simulink model "model_report_gutman"  (R2018b)
settings: Solver=FixedStepAuto  StartTime=0.0  StopTime=10  FixedStep=Ts/100  RelTol=1e-3
StopFcn:
  | %figure;plot(true_position.Data(:,1),true_position.Data(:,2))
values from neighbouring files (symbols this model uses):
  b = 1.115    [report_gutman.m]
  bike_params = [g h b a lambda m]    [report_gutman.m]
  IMU_height = 0.45    [report_gutman.m]
  initial_roll = deg2rad(2)    [report_gutman.m]
  initial_rollrate = deg2rad(2)    [report_gutman.m]
  lambda = deg2rad(90-24)    [report_gutman.m]
  num_tf_steering = [253.4]    [report_gutman.m]
  Ts = 0.01    [report_gutman.m]
  v = 4    [report_gutman.m]
undefined symbols (not defined in the file or in its folder): A, B, C, D, lqr_gains, velocity_lqr
libraries: simulink_extras x6, simulink x1
settings Model: Creator=maximef  LastModifiedBy=maximef

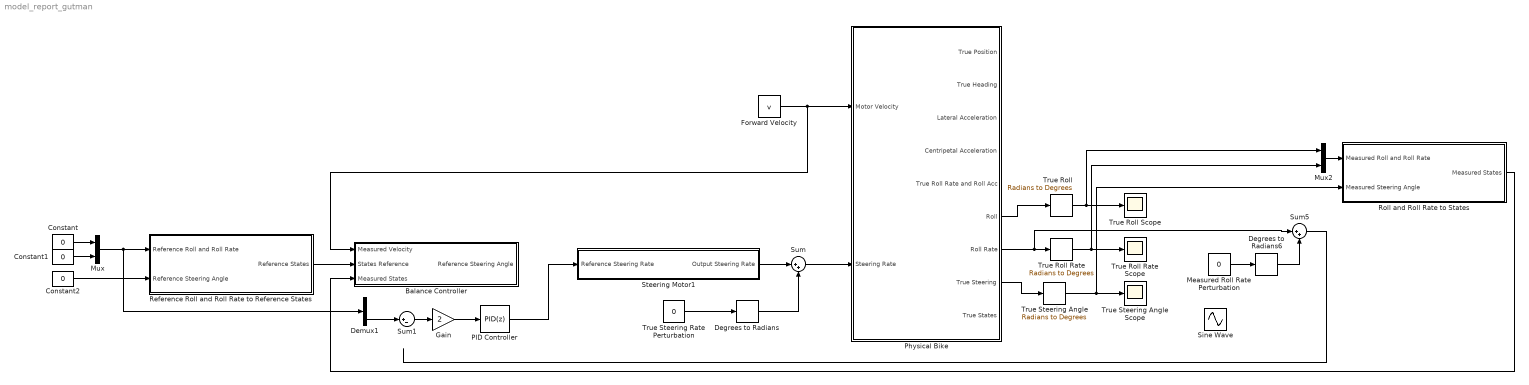
== system model_report_gutman ==
  Balance Controller : Subsystem  SystemSampleTime=Ts
  Constant : Constant  Value=0
  Constant1 : Constant  Value=0
  Constant2 : Constant  Value=0
  Degrees to Radians : simulink_extras/Transformations/Degrees to Radians
  Degrees to Radians6 : simulink_extras/Transformations/Degrees to Radians
  Demux1 : Demux  Outputs=2
  Forward Velocity : Constant  Value=v
  Gain : Gain  Gain=2
  Measured Roll Rate Perturbation : Constant  Value=0
  Mux : Mux  Inputs=2
  Mux2 : Mux  Inputs=2
  PID Controller : simulink/Continuous/PID Controller  Controller=PID  Form=Ideal  TimeDomain=Discrete-time  SampleTime=Ts  IntegratorMethod=Trapezoidal  FilterMethod=Forward Euler  ControllerParametersSource=internal  P=2.5117  I=1.5431  D=0.0750  UseFilter=off  N=5  TunerSelectOption=Transfer Function Based (PID Tuner App)  InitialConditionSource=internal  InitialConditionForIntegrator=0  InitialConditionForFilter=0  DifferentiatorICPrevScaledInput=0  ExternalReset=none  TrackingMode=off  Kt=1  LimitOutput=off  UpperSaturationLimit=inf  LowerSaturationLimit=-inf  LinearizeAsGain=on  AntiWindupMode=none  Kb=1  POutMin=[]  POutMax=[]  IOutMin=[]  IOutMax=[]  DOutMin=[]  DOutMax=[]  NOutMin=[]  NOutMax=[]  SumOutMin=[]  SumOutMax=[]  SaturationOutMin=[]  SaturationOutMax=[]  PParamMin=[]  PParamMax=[]  IParamMin=[]  IParamMax=[]  DParamMin=[]  DParamMax=[]  NParamMin=[]  NParamMax=[]  KbParamMin=[]  KbParamMax=[]  KtParamMin=[]  KtParamMax=[]  KbOutMin=[]  KbOutMax=[]  KtOutMin=[]  KtOutMax=[]  IntegratorOutMin=[]  IntegratorOutMax=[]  FilterOutMin=[]  FilterOutMax=[]  SumI1OutMin=[]  SumI1OutMax=[]  SumI2OutMin=[]  SumI2OutMax=[]  SumI3OutMin=[]  SumI3OutMax=[]  SumI4OutMin=[]  SumI4OutMax=[]  SumDOutMin=[]  SumDOutMax=[]  DifferentiatorOutMin=[]  DifferentiatorOutMax=[]  FilterDiffOutCoefMin=[]  FilterDiffOutCoefMax=[]  ReciprocalOutMin=[]  ReciprocalOutMax=[]  SumDenOutMin=[]  SumDenOutMax=[]  SumNumOutMin=[]  SumNumOutMax=[]  DivideOutMin=[]  DivideOutMax=[]  IntegratorContinuousStateAttributes=''  IntegratorStateMustResolveToSignalObject=off  IntegratorRTWStateStorageClass=Auto  FilterContinuousStateAttributes=''  FilterStateMustResolveToSignalObject=off  FilterRTWStateStorageClass=Auto  ParallelPVariant=Passthrough  IdealPVariant=InternalParameters  IVariant=InternalParameters  DVariant=InternalParameters  IntegratorVariant=Discrete  SatVariant=Disabled  AWVariant=Passthrough  PCopyVariant=Disabled  TRVariant=Disabled  FdbkBlocksVariant=Forward  IdealPFdbkVariant=Disabled  SatFdbkVariant=Disabled  DerivativeFilterVariant=Differentiator  NVariant=Passthrough  NCopyVariant=Disabled_SignalSpec  FilterICVariant=InternalICsDifferentiator  IntegratorICVariant=InternalICs  ExternalResetVariant=Disabled  TRSumVariant=Passthrough  SumFdbkVariant=Disabled  SumVariant=Sum_PID
  Physical Bike : Subsystem
  Reference Roll and Roll Rate to Reference States : Subsystem
  Roll and Roll Rate to States : Subsystem
  Sine Wave : Sin  Amplitude=2  Frequency=2*pi*40  SampleTime=Ts
  Steering Motor1 : Subsystem
  Sum : Sum  Inputs=|++
  Sum1 : Sum  Inputs=|+-
  Sum5 : Sum  Inputs=|++
  True Roll : simulink_extras/Transformations/Radians to Degrees
  True Roll Rate : simulink_extras/Transformations/Radians to Degrees
  True Roll Rate Scope : Scope
  True Roll Scope : Scope
  True Steering Angle : simulink_extras/Transformations/Radians to Degrees
  True Steering Angle Scope : Scope
  True Steering Rate Perturbation : Constant  Value=0
  wires:
  True Roll Rate/1 -> True Roll Rate Scope/1, Mux2/2
  Measured Roll Rate Perturbation/1 -> Degrees to Radians6/1
  Physical Bike/6(Roll) -> True Roll/1
  Sum/1 -> Physical Bike/2(Steering Rate)
  True Steering Angle/1 -> Roll and Roll Rate to States/2(Measured Steering Angle), True Steering Angle Scope/1
  Constant/1 -> Mux/1
  True Steering Rate Perturbation/1 -> Degrees to Radians/1
  Forward Velocity/1 -> Balance Controller/1(Measured Velocity), Physical Bike/1(Motor Velocity)
  Degrees to Radians/1 -> Sum/2
  True Roll/1 -> Mux2/1, True Roll Scope/1
  Degrees to Radians6/1 -> Sum5/2
  Constant1/1 -> Mux/2
  Physical Bike/8(True Steering) -> True Steering Angle/1
  Physical Bike/7(Roll Rate) -> Sum5/1, True Roll Rate/1
  Sum1/1 -> Gain/1
  Sum5/1 -> ?
  Reference Roll and Roll Rate to Reference States/1(Reference States) -> Balance Controller/2(States Reference)
  Constant2/1 -> Reference Roll and Roll Rate to Reference States/2(Reference Steering Angle)
  Demux1/2 -> Sum1/1
  Gain/1 -> PID Controller/1
  Mux/1 -> Demux1/1, Reference Roll and Roll Rate to Reference States/1(Reference Roll and Roll Rate)
  Mux2/1 -> Roll and Roll Rate to States/1(Measured Roll and Roll Rate)
  Roll and Roll Rate to States/1(Measured States) -> Balance Controller/3(Measured States)
  PID Controller/1 -> Steering Motor1/1(Reference Steering Rate)
  Steering Motor1/1(Output Steering Rate) -> Sum/1

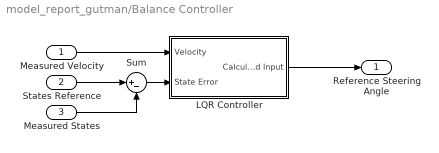
== system model_report_gutman/Balance Controller ==
  Measured Velocity : Inport
  States Reference : Inport  Port=2
  Measured States : Inport  Port=3
  LQR Controller : Subsystem  TreatAsAtomicUnit=on  SystemSampleTime=Ts
  Sum : Sum  Inputs=|+-
  Reference Steering Angle : Outport
  wires:
  Sum/1 -> LQR Controller/2(State Error)
  Measured States/1 -> Sum/2
  LQR Controller/1(Calculated Input) -> Reference Steering Angle/1
  Measured Velocity/1 -> LQR Controller/1(Velocity)
  States Reference/1 -> Sum/1

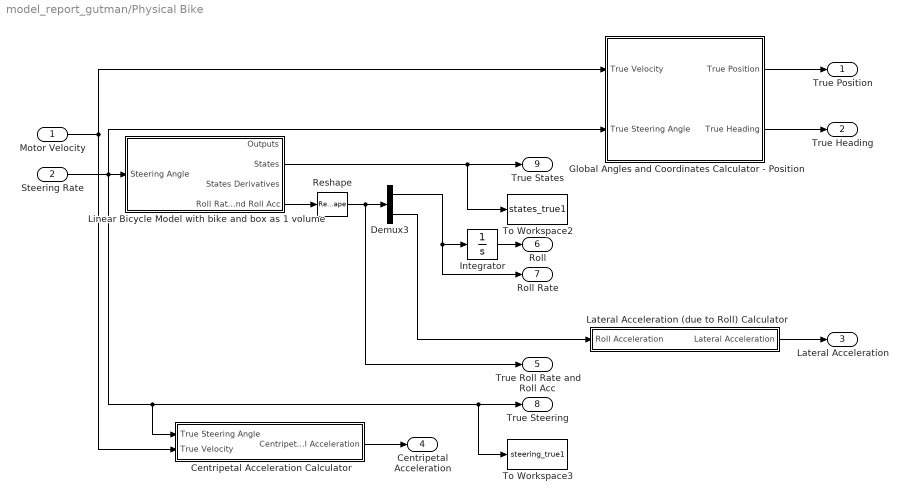
== system model_report_gutman/Physical Bike ==
  Motor Velocity : Inport
  Steering Rate : Inport  Port=2
  Centripetal Acceleration Calculator : Subsystem
  Demux3 : Demux  Outputs=2
  Global Angles and Coordinates Calculator - Position : Subsystem  SystemSampleTime=Ts
  Integrator : Integrator  InitialCondition=initial_roll
  Lateral Acceleration (due to Roll) Calculator : Subsystem
  Linear Bicycle Model with bike and box as 1 volume : Subsystem
  Reshape : Reshape
  To Workspace2 : ToWorkspace  VariableName=states_true1  SaveFormat=Timeseries  SampleTime=-1
  To Workspace3 : ToWorkspace  VariableName=steering_true1  SaveFormat=Timeseries  SampleTime=-1
  True Position : Outport
  True Heading : Outport  Port=2
  Lateral Acceleration : Outport  Port=3
  Centripetal Acceleration : Outport  Port=4
  True Roll Rate and Roll Acc : Outport  Port=5
  Roll : Outport  Port=6
  Roll Rate : Outport  Port=7
  True Steering : Outport  Port=8
  True States : Outport  Port=9
  wires:
  Steering Rate/1 -> Global Angles and Coordinates Calculator - Position/2(True Steering Angle), To Workspace3/1, True Steering/1, Centripetal Acceleration Calculator/1(True Steering Angle), Linear Bicycle Model with bike and box as 1 volume/1(Steering Angle)
  Centripetal Acceleration Calculator/1(Centripetal Acceleration) -> Centripetal Acceleration/1
  Demux3/2 -> Lateral Acceleration (due to Roll) Calculator/1(Roll Acceleration)
  Lateral Acceleration (due to Roll) Calculator/1(Lateral Acceleration) -> Lateral Acceleration/1
  Linear Bicycle Model with bike and box as 1 volume/2(States) -> To Workspace2/1, True States/1
  Demux3/1 -> Integrator/1, Roll Rate/1
  Reshape/1 -> True Roll Rate and Roll Acc/1, Demux3/1
  Linear Bicycle Model with bike and box as 1 volume/4(Roll Rate and Roll Acc) -> Reshape/1
  Motor Velocity/1 -> Centripetal Acceleration Calculator/2(True Velocity), Global Angles and Coordinates Calculator - Position/1(True Velocity)
  Global Angles and Coordinates Calculator - Position/1(True Position) -> True Position/1
  Global Angles and Coordinates Calculator - Position/2(True Heading) -> True Heading/1
  Integrator/1 -> Roll/1

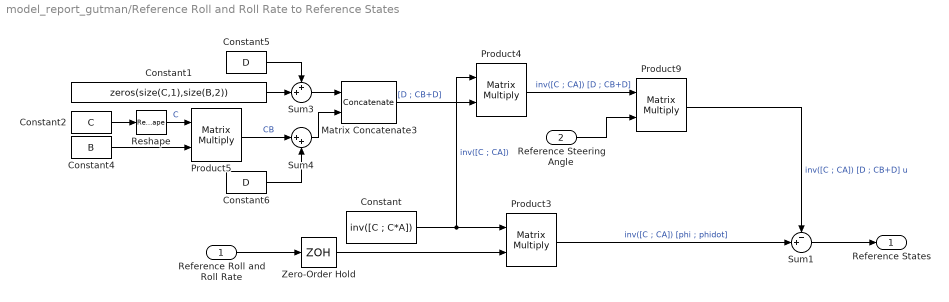
== system model_report_gutman/Reference Roll and Roll Rate to Reference States ==
  Reference Roll and Roll Rate : Inport
  Reference Steering Angle : Inport  Port=2
  Constant : Constant  Value=inv([C ; C*A])
  Constant1 : Constant  Value=zeros(size(C,1),size(B,2))
  Constant2 : Constant  Value=C
  Constant4 : Constant  Value=B
  Constant5 : Constant  Value=D
  Constant6 : Constant  Value=D
  Matrix Concatenate3 : Concatenate  Mode=Multidimensional array
  Product{3..5,9} (4 alike) : Product  SCDEnableBlockLinearizationSpecification=on  Multiplication=Matrix(*)
  Reshape : Reshape  OutputDimensionality=Customize  OutputDimensions=[size(C,1),size(C,2)]
  Sum1 : Sum  Inputs=-+|
  Sum3 : Sum  Inputs=++|
  Sum4 : Sum  Inputs=|++
  Zero-Order Hold : ZeroOrderHold  SampleTime=Ts
  Reference States : Outport
  wires:
  Constant2/1 -> Reshape/1
  Constant/1 -> Product4/1, Product3/1  "inv([C ; CA])"
  Reference Roll and Roll Rate/1 -> Zero-Order Hold/1
  Product3/1 -> Sum1/2  "inv([C ; CA]) [phi ; phidot]"
  Matrix Concatenate3/1 -> Product4/2  "[D ; CB+D]"
  Product5/1 -> Sum4/1  "CB"
  Constant4/1 -> Product5/2
  Constant1/1 -> Sum3/2
  Product4/1 -> Product9/1  "inv([C ; CA]) [D ; CB+D]"
  Reference Steering Angle/1 -> Product9/2
  Product9/1 -> Sum1/1  "inv([C ; CA]) [D ; CB+D] u"
  Sum1/1 -> Reference States/1
  Zero-Order Hold/1 -> Product3/2
  Constant6/1 -> Sum4/2
  Constant5/1 -> Sum3/1
  Sum4/1 -> Matrix Concatenate3/2
  Sum3/1 -> Matrix Concatenate3/1
  Reshape/1 -> Product5/1  "C"

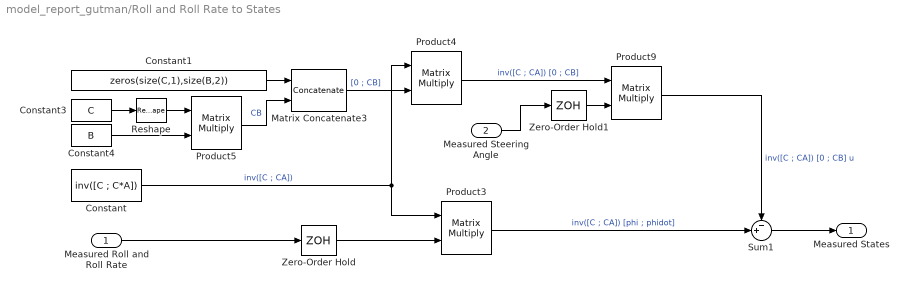
== system model_report_gutman/Roll and Roll Rate to States ==
  Measured Roll and Roll Rate : Inport
  Measured Steering Angle : Inport  Port=2
  Constant : Constant  Value=inv([C ; C*A])
  Constant1 : Constant  Value=zeros(size(C,1),size(B,2))
  Constant3 : Constant  Value=C
  Constant4 : Constant  Value=B
  Matrix Concatenate3 : Concatenate  Mode=Multidimensional array
  Product{3..5,9} (4 alike) : Product  SCDEnableBlockLinearizationSpecification=on  Multiplication=Matrix(*)
  Reshape : Reshape  OutputDimensionality=Row vector (2-D)
  Sum1 : Sum  Inputs=-+|
  Zero-Order Hold : ZeroOrderHold  SampleTime=Ts
  Zero-Order Hold1 : ZeroOrderHold  SampleTime=Ts
  Measured States : Outport
  wires:
  Constant/1 -> Product3/1, Product4/1  "inv([C ; CA])"
  Measured Roll and Roll Rate/1 -> Zero-Order Hold/1
  Product3/1 -> Sum1/2  "inv([C ; CA]) [phi ; phidot]"
  Matrix Concatenate3/1 -> Product4/2  "[0 ; CB]"
  Product5/1 -> Matrix Concatenate3/2  "CB"
  Constant1/1 -> Matrix Concatenate3/1
  Product4/1 -> Product9/1  "inv([C ; CA]) [0 ; CB]"
  Measured Steering Angle/1 -> Zero-Order Hold1/1
  Product9/1 -> Sum1/1  "inv([C ; CA]) [0 ; CB] u"
  Sum1/1 -> Measured States/1
  Zero-Order Hold/1 -> Product3/2
  Constant3/1 -> Reshape/1
  Constant4/1 -> Product5/2
  Reshape/1 -> Product5/1
  Zero-Order Hold1/1 -> Product9/2

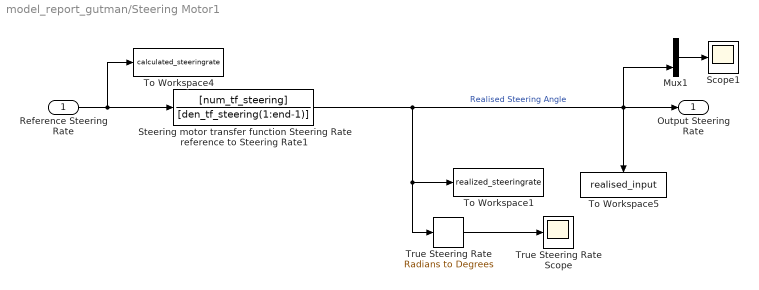
== system model_report_gutman/Steering Motor1 ==
  Reference Steering Rate : Inport
  Mux1 : Mux  Inputs=2
  Scope1 : Scope
  Steering motor transfer function Steering Rate reference to Steering Rate1 : TransferFcn  Numerator=[num_tf_steering]  Denominator=[den_tf_steering(1:end-1)]
  To Workspace1 : ToWorkspace  VariableName=realized_steeringrate  SaveFormat=Timeseries  SampleTime=Ts
  To Workspace4 : ToWorkspace  VariableName=calculated_steeringrate  SaveFormat=Timeseries  SampleTime=Ts
  To Workspace5 : ToWorkspace  VariableName=realised_input  SaveFormat=Timeseries  SampleTime=Ts
  True Steering Rate : simulink_extras/Transformations/Radians to Degrees
  True Steering Rate Scope : Scope
  Output Steering Rate : Outport
  wires:
  Mux1/1 -> Scope1/1
  Steering motor transfer function Steering Rate reference to Steering Rate1/1 -> Output Steering Rate/1, Mux1/2, To Workspace5/1, True Steering Rate/1, To Workspace1/1  "Realised Steering Angle"
  True Steering Rate/1 -> True Steering Rate Scope/1
  Reference Steering Rate/1 -> To Workspace4/1, Steering motor transfer function Steering Rate reference to Steering Rate1/1

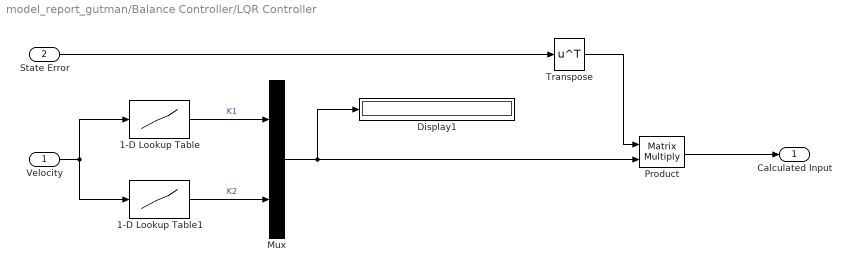
== system model_report_gutman/Balance Controller/LQR Controller ==
  Velocity : Inport
  State Error : Inport  Port=2
  1-D Lookup Table : Lookup_n-D  NumberOfTableDimensions=1  BreakpointsForDimension1=velocity_lqr  BreakpointsForDimension2=velocity_lqr  BreakpointsForDimension3=velocity_lqr  BreakpointsForDimension4=velocity_lqr  Table=lqr_gains(:,2)  InternalRulePriority=Speed  RndMeth=Simplest  InputSameDT=on
  1-D Lookup Table1 : Lookup_n-D  NumberOfTableDimensions=1  BreakpointsForDimension1=velocity_lqr  BreakpointsForDimension2=velocity_lqr  BreakpointsForDimension3=velocity_lqr  BreakpointsForDimension4=velocity_lqr  Table=lqr_gains(:,3)  InternalRulePriority=Speed  RndMeth=Simplest  InputSameDT=on
  Display1 : Display
  Mux : Mux  Inputs=2
  Product : Product  Multiplication=Matrix(*)
  Transpose : Math  Operator=transpose  SaturateOnIntegerOverflow=on
  Calculated Input : Outport
  wires:
  1-D Lookup Table/1 -> Mux/1  "K1"
  1-D Lookup Table1/1 -> Mux/2  "K2"
  Velocity/1 -> 1-D Lookup Table1/1, 1-D Lookup Table/1
  Mux/1 -> Product/2, Display1/1
  Transpose/1 -> Product/1
  Product/1 -> Calculated Input/1
  State Error/1 -> Transpose/1

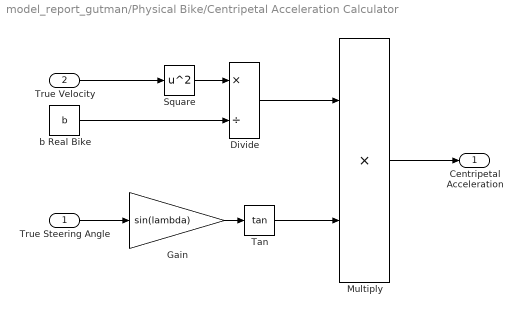
== system model_report_gutman/Physical Bike/Centripetal Acceleration Calculator ==
  True Steering Angle : Inport
  True Velocity : Inport  Port=2
  Divide : Product  Inputs=*/
  Gain : Gain  Gain=sin(lambda)
  Multiply : Product
  Square : Math  Operator=square  SaturateOnIntegerOverflow=on
  Tan : Trigonometry  Operator=tan
  b Real Bike : Constant  Value=b
  Centripetal Acceleration : Outport
  wires:
  True Velocity/1 -> Square/1
  Square/1 -> Divide/1
  b Real Bike/1 -> Divide/2
  True Steering Angle/1 -> Gain/1
  Divide/1 -> Multiply/1
  Tan/1 -> Multiply/2
  Multiply/1 -> Centripetal Acceleration/1
  Gain/1 -> Tan/1

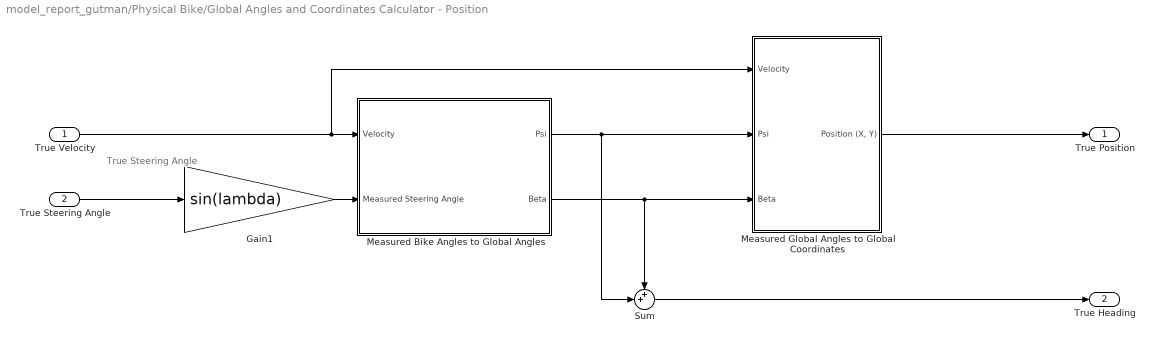
== system model_report_gutman/Physical Bike/Global Angles and Coordinates Calculator - Position ==
  note: True Steering
      | Angle
  True Velocity : Inport
  True Steering Angle : Inport  Port=2
  Gain1 : Gain  Gain=sin(lambda)
  Measured Bike Angles to Global Angles : Subsystem
  Measured Global Angles to Global Coordinates : Subsystem
  Sum : Sum  Inputs=++|
  True Position : Outport
  True Heading : Outport  Port=2
  wires:
  Measured Bike Angles to Global Angles/1(Psi) -> Sum/2, Measured Global Angles to Global Coordinates/2(Psi)
  Gain1/1 -> Measured Bike Angles to Global Angles/2(Measured Steering Angle)
  Sum/1 -> True Heading/1
  Measured Bike Angles to Global Angles/2(Beta) -> Sum/1, Measured Global Angles to Global Coordinates/3(Beta)
  Measured Global Angles to Global Coordinates/1("Position (X, Y)") -> True Position/1
  True Velocity/1 -> Measured Global Angles to Global Coordinates/1(Velocity), Measured Bike Angles to Global Angles/1(Velocity)
  True Steering Angle/1 -> Gain1/1

== system model_report_gutman/Physical Bike/Lateral Acceleration (due to Roll) Calculator ==
  Roll Acceleration : Inport
  Constant3 : Constant  Value=IMU_height
  Multiply : Product
  Lateral Acceleration : Outport
  wires:
  Multiply/1 -> Lateral Acceleration/1
  Constant3/1 -> Multiply/1
  Roll Acceleration/1 -> Multiply/2

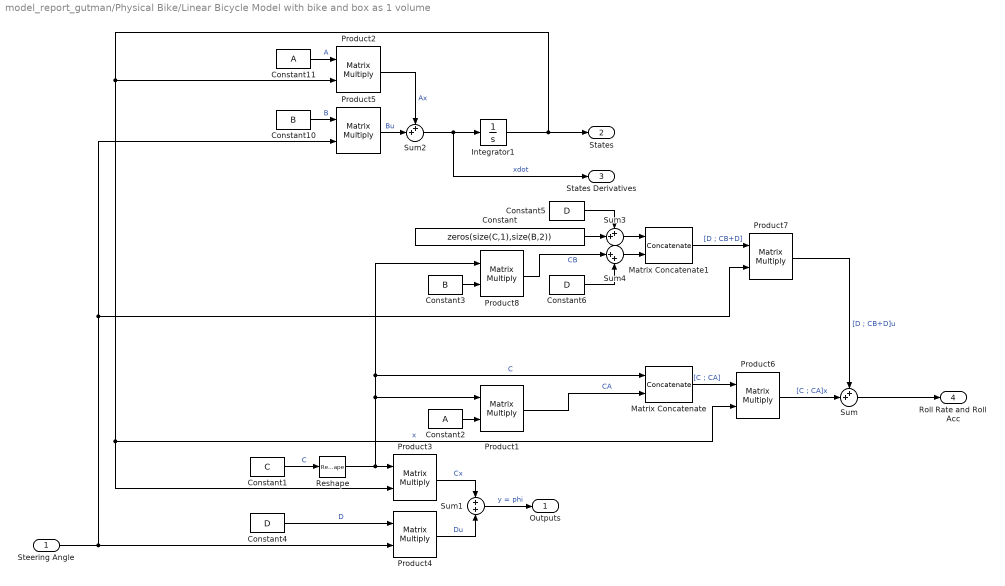
== system model_report_gutman/Physical Bike/Linear Bicycle Model with bike and box as 1 volume ==
  Steering Angle : Inport
  Constant : Constant  Value=zeros(size(C,1),size(B,2))
  Constant1 : Constant  Value=C
  Constant10 : Constant  Value=B
  Constant11 : Constant  Value=A
  Constant2 : Constant  Value=A
  Constant3 : Constant  Value=B
  Constant4 : Constant  Value=D
  Constant5 : Constant  Value=D
  Constant6 : Constant  Value=D
  Integrator1 : Integrator  InitialCondition=[C ; C*A]\[initial_rollrate ; 0]
  Matrix Concatenate : Concatenate  Mode=Multidimensional array
  Matrix Concatenate1 : Concatenate  Mode=Multidimensional array
  Product{1..8} (8 alike) : Product  SCDEnableBlockLinearizationSpecification=on  Multiplication=Matrix(*)
  Reshape : Reshape  OutputDimensionality=Customize  OutputDimensions=[size(C,1),size(C,2)]
  Sum : Sum  Inputs=++|
  Sum1 : Sum
  Sum2 : Sum  Inputs=++|
  Sum3 : Sum  Inputs=++|
  Sum4 : Sum  Inputs=|++
  Outputs : Outport
  States : Outport  Port=2
  States Derivatives : Outport  Port=3
  Roll Rate and Roll Acc : Outport  Port=4
  wires:
  Reshape/1 -> Product3/1, Product8/1, Matrix Concatenate/1, Product1/1  "C"
  Sum/1 -> Roll Rate and Roll Acc/1
  Constant1/1 -> Reshape/1  "C"
  Matrix Concatenate/1 -> Product6/1  "[C ; CA]"
  Product5/1 -> Sum2/2  "Bu"
  Matrix Concatenate1/1 -> Product7/1  "[D ; CB+D]"
  Constant11/1 -> Product2/1  "A"
  Constant3/1 -> Product8/2
  Product6/1 -> Sum/2  "[C ; CA]x"
  Sum2/1 -> Integrator1/1, States Derivatives/1  "xdot"
  Product2/1 -> Sum2/1  "Ax"
  Product1/1 -> Matrix Concatenate/2  "CA"
  Product8/1 -> Sum4/1  "CB"
  Integrator1/1 -> Product2/2, Product6/2, Product3/2, States/1  "x"
  Sum1/1 -> Outputs/1  "y = phi"
  Constant2/1 -> Product1/2
  Product7/1 -> Sum/1  "[D ; CB+D]u"
  Constant10/1 -> Product5/1  "B"
  Steering Angle/1 -> Product4/2, Product5/2, Product7/2
  Product4/1 -> Sum1/2  "Du"
  Product3/1 -> Sum1/1  "Cx"
  Constant4/1 -> Product4/1  "D"
  Sum3/1 -> Matrix Concatenate1/1
  Constant/1 -> Sum3/2
  Constant5/1 -> Sum3/1
  Sum4/1 -> Matrix Concatenate1/2
  Constant6/1 -> Sum4/2

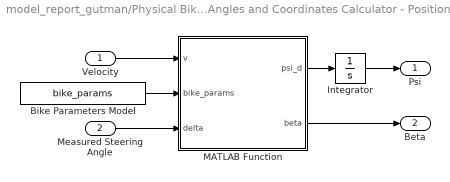
== system model_report_gutman/Physical Bike/Global Angles and Coordinates Calculator - Position/Measured Bike Angles to Global Angles ==
  Velocity : Inport
  Measured Steering Angle : Inport  Port=2
  " Bike Parameters Model " : Constant  Value=bike_params
  Integrator : Integrator
  MATLAB Function : MATLAB Function  TreatAsAtomicUnit=on
  Psi : Outport
  Beta : Outport  Port=2
  wires:
  MATLAB Function/2(beta) -> Beta/1
  MATLAB Function/1(psi_d) -> Integrator/1
  Integrator/1 -> Psi/1
  " Bike Parameters Model "/1 -> MATLAB Function/2(bike_params)
  Measured Steering Angle/1 -> MATLAB Function/3(delta)
  Velocity/1 -> MATLAB Function/1(v)

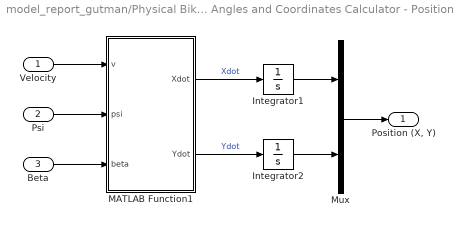
== system model_report_gutman/Physical Bike/Global Angles and Coordinates Calculator - Position/Measured Global Angles to Global Coordinates ==
  Velocity : Inport
  Psi : Inport  Port=2
  Beta : Inport  Port=3
  Integrator1 : Integrator
  Integrator2 : Integrator
  MATLAB Function1 : MATLAB Function  TreatAsAtomicUnit=on
  Mux : Mux  Inputs=2
  "Position (X, Y)" : Outport
  wires:
  MATLAB Function1/2(Ydot) -> Integrator2/1  "Ydot"
  MATLAB Function1/1(Xdot) -> Integrator1/1  "Xdot"
  Psi/1 -> MATLAB Function1/2(psi)
  Beta/1 -> MATLAB Function1/3(beta)
  Velocity/1 -> MATLAB Function1/1(v)
  Integrator2/1 -> Mux/2
  Integrator1/1 -> Mux/1
  Mux/1 -> "Position (X, Y)"/1

== matlab function model_report_gutman/Physical Bike/Global Angles and Coordinates Calculator - Position/Measured Bike Angles to Global Angles/MATLAB Function ==
  data: v input; bike_params input; delta input; psi_d output; beta output
function [psi_d, beta]  = fcn(v, bike_params, delta)

b = bike_params(3);
a = bike_params(4);

beta = atan((a / (b)) * tan(delta));
psi_d = (v / a) * sin(beta);

== matlab function model_report_gutman/Physical Bike/Global Angles and Coordinates Calculator - Position/Measured Global Angles to Global Coordinates/MATLAB Function1 ==
  data: v input; psi input; Xdot output; beta input; Ydot output
function [Xdot, Ydot]  = fcn(v, psi, beta)

Xdot = v * cos(psi + beta);
Ydot = v * sin(psi + beta);
